simulink model "sheme_4_5"  (R2018a)
settings: Solver=ode45  StartTime=0.0  StopTime=40  RelTol=1e-3  EnableMultiTasking=on
settings Model: Creator=stud507ikt  LastModifiedBy=Asus
settings DataIOCC: LimitDataPoints=on  SaveFormat=Array
settings OptimizationCC: LifeSpan=inf
settings DebuggingCC: SolverPrmCheckMsg=warning  SFUnexpectedBacktrackingDiag=warning  SFNoUnconditionalDefaultTransitionDiag=warning  SFExecutionAtInitializationDiag=none
settings HardwareCC: ProdBitPerPointer=32  ProdBitPerSizeT=32  ProdBitPerPtrDiffT=32  ProdLargestAtomicFloat=None  ProdIntDivRoundTo=Undefined  ProdEndianess=Unspecified  ProdWordSize=32  ProdHWDeviceType=32-bit Generic
settings ModelReferenceCC: PropagateSignalLabelsOutOfModel=off
settings CodeAppCC: StateflowObjectComments=on
settings GRTTargetCC: TargetLangStandard=C89/C90 (ANSI)  GeneratePreprocessorConditionals=Disable all
settings ConfigComp: CovMetricSettings=dw  CovHtmlReporting=on  CovSaveCumulativeToWorkspaceVar=on  CovSaveSingleToWorkspaceVar=on  CovExternalEMLEnable=off  CovSFcnEnable=off

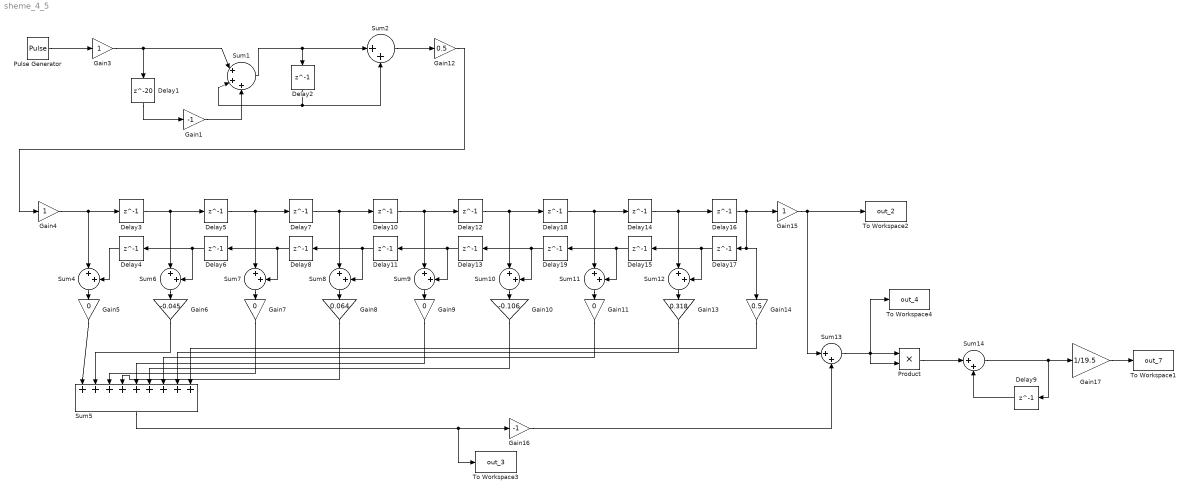
== system sheme_4_5 ==
  Delay1 : Delay  DelayLength=20  InitialCondition=0  InputProcessing=Inherited
  Delay{2..19} (18 alike) : Delay  DelayLength=1  InitialCondition=0  InputProcessing=Inherited
  Gain1 : Gain  Gain=-1
  Gain10 : Gain  Gain=-0.106
  Gain{5,7,9,11} (4 alike) : Gain  Gain=0
  Gain12 : Gain  Gain=0.5
  Gain13 : Gain  Gain=0.318
  Gain14 : Gain  Gain=0.5
  Gain15 : Gain
  Gain16 : Gain  Gain=-1
  Gain17 : Gain  Gain=1/19.5
  Gain3 : Gain
  Gain4 : Gain
  Gain6 : Gain  Gain=-0.045
  Gain8 : Gain  Gain=0.064
  Product : Product
  Pulse Generator : DiscretePulseGenerator  Period=10000
  Sum1 : Sum  Inputs=|+++
  Sum{2,4,6..14} (11 alike) : Sum  Inputs=|++
  Sum5 : Sum  Inputs=|+++++++++
  To Workspace1 : ToWorkspace  VariableName=out_7  SampleTime=-1
  To Workspace2 : ToWorkspace  VariableName=out_2  SampleTime=-1
  To Workspace3 : ToWorkspace  VariableName=out_3  SampleTime=-1
  To Workspace4 : ToWorkspace  VariableName=out_4  SampleTime=-1
  wires:
  Delay1/1 -> Gain1/1
  Gain1/1 -> Sum1/3
  Delay2/1 -> Sum1/2, Sum2/2
  Sum1/1 -> Sum2/1, Delay2/1
  Sum2/1 -> Gain12/1
  Gain3/1 -> Delay1/1, Sum1/1
  Gain4/1 -> Sum4/1, Delay3/1
  Sum4/1 -> Gain5/1
  Gain5/1 -> Sum5/1
  Delay4/1 -> Sum4/2
  Sum6/1 -> Gain6/1
  Delay6/1 -> Delay4/1, Sum6/2
  Delay3/1 -> Sum6/1, Delay5/1
  Delay5/1 -> Sum7/1, Delay7/1
  Delay8/1 -> Delay6/1, Sum7/2
  Sum7/1 -> Gain7/1
  Delay7/1 -> Sum8/1, Delay10/1
  Sum8/1 -> Gain8/1
  Delay13/1 -> Delay11/1, Sum9/2
  Delay11/1 -> Delay8/1, Sum8/2
  Delay10/1 -> Sum9/1, Delay12/1
  Sum9/1 -> Gain9/1
  Sum12/1 -> Gain13/1
  Delay14/1 -> Sum12/1, Delay16/1
  Delay15/1 -> Delay19/1, Sum11/2
  Delay17/1 -> Delay15/1, Sum12/2
  Sum11/1 -> Gain11/1
  Delay19/1 -> Delay13/1, Sum10/2
  Delay18/1 -> Sum11/1, Delay14/1
  Delay12/1 -> Sum10/1, Delay18/1
  Sum10/1 -> Gain10/1
  Delay16/1 -> Gain15/1, Gain14/1, Delay17/1
  Gain6/1 -> Sum5/2
  Gain7/1 -> Sum5/3
  Gain8/1 -> Sum5/4
  Gain9/1 -> Sum5/5
  Gain10/1 -> Sum5/6
  Gain11/1 -> Sum5/7
  Gain13/1 -> Sum5/8
  Gain14/1 -> Sum5/9
  Pulse Generator/1 -> Gain3/1
  Gain12/1 -> Gain4/1
  Sum5/1 -> To Workspace3/1, Gain16/1
  Gain16/1 -> Sum13/2
  Gain15/1 -> Sum13/1, To Workspace2/1
  Sum13/1 -> To Workspace4/1, Product/2, Product/1
  Delay9/1 -> Sum14/2
  Sum14/1 -> Delay9/1, Gain17/1
  Product/1 -> Sum14/1
  Gain17/1 -> To Workspace1/1
